simulink model "ex5_2"  (R2020a)
settings: Solver=VariableStepAuto  StartTime=0.0  StopTime=10.0  RelTol=1e-3
settings Model: Creator=반달  LastModifiedBy=반달

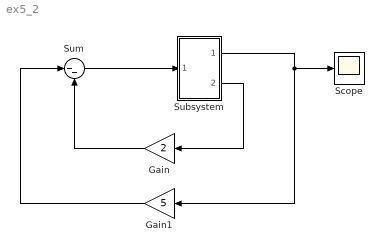
== system ex5_2 ==
  Gain : Gain  Gain=2
  Gain1 : Gain  Gain=5
  Scope : Scope
  Subsystem : Subsystem
  Sum : Sum  Inputs=|--
  wires:
  Gain/1 -> Sum/2
  Gain1/1 -> Sum/1
  Subsystem/1(Out1) -> Gain1/1, Scope/1
  Sum/1 -> Subsystem/1(In1)
  Subsystem/2(Out2) -> Gain/1

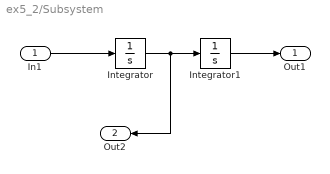
== system ex5_2/Subsystem ==
  In1 : Inport
  Integrator : Integrator
  Integrator1 : Integrator  InitialCondition=4
  Out1 : Outport
  Out2 : Outport  Port=2
  wires:
  Integrator/1 -> Out2/1, Integrator1/1
  In1/1 -> Integrator/1
  Integrator1/1 -> Out1/1
